simulink model "single_drone_simulink"  (R2022a)
settings: Solver=VariableStepAuto  StartTime=0.0  StopTime=20  RelTol=1e-3
undefined symbols (not defined in the file): A_dual, B_dual, C_dual, D_dual, K_dual
libraries: SignalEditorBlockLib x1, simulink x1
settings Model: Creator=blume  LastModifiedBy=blume

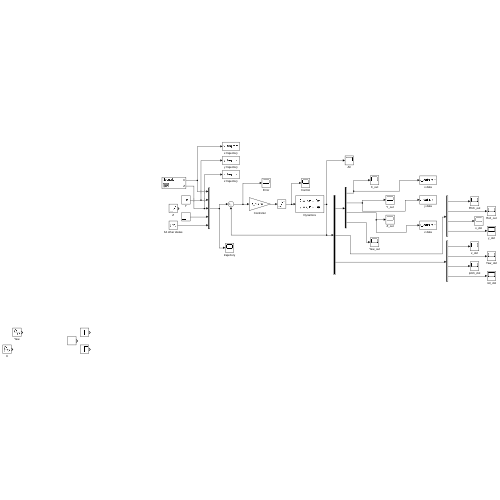
[thumbnail: Simulink's stored preview of the top-level diagram]
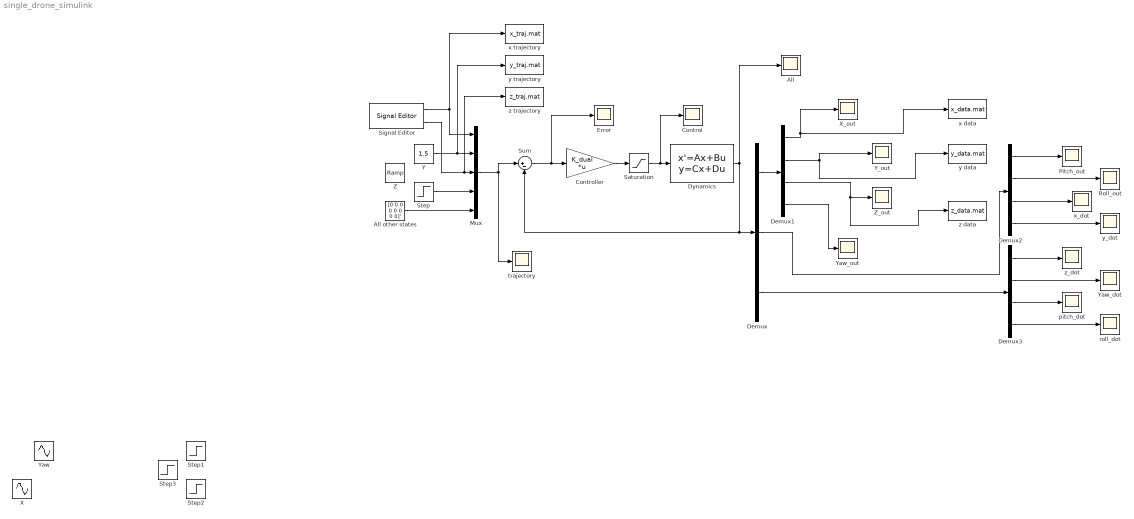
== system single_drone_simulink ==
  All : Scope
  All other states : Constant  Value=[0 0 0 0 0 0 0 0]'
  Control : Scope
  Controller : Gain  Gain=K_dual  Multiplication=Matrix(K*u)
  Demux : Demux  Outputs=3
  Demux1 : Demux
  Demux2 : Demux
  Demux3 : Demux
  Dynamics : StateSpace  A=A_dual  B=B_dual  C=C_dual  D=D_dual  InitialCondition=0
  Error : Scope
  Mux : Mux  Inputs=5
  Pitch_out : Scope
  Roll_out : Scope
  Saturation : Saturate  UpperLimit=7000  LowerLimit=-6000
  Signal Editor : SignalEditorBlockLib/Signal Editor  FileName=x_z.mat  ActiveScenario=Scenario  ActiveSignal=X  IsBus=off  OutputBusObjectStr=Bus: BusObject  SampleTime=0  Interpolate=off  ZeroCross=off  OutputAfterFinalValue=Setting to zero  Unit=inherit  PreserveSignalName=on
  Step : Step  Time=4  After=pi/4  SampleTime=0
  Step1 : Step  Time=10  After=0  SampleTime=0
  Step2 : Step  Time=0  After=0  SampleTime=0
  Step3 : Step  Time=2  After=2  SampleTime=0
  Sum : Sum  Inputs=|+-
  X : Sin  Frequency=0.25  SampleTime=0
  X_out : Scope
  Y : Constant  Value=1.5
  Y_out : Scope
  Yaw : Sin  Frequency=0.25  SampleTime=0
  Yaw_dot : Scope
  Yaw_out : Scope
  Z : simulink/Sources/Ramp  slope=1  start=0  InitialOutput=0
  Z_out : Scope
  pitch_dot : Scope
  roll_dot : Scope
  trajectory : Scope
  x data : ToFile  Filename=x_data.mat  MatrixName=x  SaveFormat=Timeseries
  x trajectory : ToFile  Filename=x_traj.mat  MatrixName=x_traj  SaveFormat=Timeseries
  x_dot : Scope
  y data : ToFile  Filename=y_data.mat  MatrixName=y  SaveFormat=Timeseries
  y trajectory : ToFile  Filename=y_traj.mat  MatrixName=y_traj  SaveFormat=Timeseries
  y_dot : Scope
  z data : ToFile  Filename=z_data.mat  MatrixName=z  SaveFormat=Timeseries
  z trajectory : ToFile  Filename=z_traj.mat  MatrixName=z_traj  SaveFormat=Timeseries
  z_dot : Scope
  wires:
  Mux/1 -> Sum/1, trajectory/1
  Sum/1 -> Error/1, Controller/1
  Dynamics/1 -> Sum/2, Demux/1, All/1
  Controller/1 -> Saturation/1
  Demux/1 -> Demux1/1
  Demux1/1 -> X_out/1, x data/1
  Demux1/2 -> y data/1, Y_out/1
  Demux1/3 -> z data/1, Z_out/1
  Demux1/4 -> Yaw_out/1
  All other states/1 -> Mux/5
  Demux/2 -> Demux2/1
  Demux/3 -> Demux3/1
  Demux3/1 -> z_dot/1
  Demux2/4 -> y_dot/1
  Demux2/3 -> x_dot/1
  Demux2/2 -> Roll_out/1
  Demux2/1 -> Pitch_out/1
  Demux3/2 -> Yaw_dot/1
  Demux3/3 -> pitch_dot/1
  Demux3/4 -> roll_dot/1
  Y/1 -> Mux/2, y trajectory/1
  Signal Editor/1 -> Mux/1, x trajectory/1
  Signal Editor/2 -> z trajectory/1, Mux/3
  Step/1 -> Mux/4
  Saturation/1 -> Dynamics/1, Control/1
